simulink model "ModelOfLikeTheWholeThing"  (R2017b)
settings: Solver=ode8  StartTime=0.0  StopTime=5  FixedStep=0.01  RelTol=1e-3
InitFcn:
  | ra = 4;
  | jm = 0.0000218;
  | rm = 0.7/100;
  | dsm = 62.892;
  | kt = 0.138;
  | ke = kt;
  | ms = 0.93;
  | hl = 1.5 / 100;
  | Lr = 24.1 / 100;
  | Lcm = hl / 2 + Lr;
  | ml =0.182;
  | mr = 0.085;
  | rl = 20.125 / 1000;
  | Jp =1/3 * mr * Lr^2 + 1/2*ml*rl^2 + ml * Lcm ^ 2;
  | Dp = 0.007;
  | g = 9.82;
StartFcn:
  | ra = 4;
  | jm = 0.0000218;
  | rm = 0.7/100;
  | dsm = 62.892;
  | kt = 0.138;
  | ke = kt;
  | ms = 0.93;
settings Model: Creator=labadmin  LastModifiedBy=labadmin
settings RTWCC: SystemTargetFile=sldrt.tlc  TemplateMakefile=sldrt.tmf  Description=Simulink Desktop Real-Time  RTWCompilerOptimization=on
settings CodeAppCC: MaxIdLength=95
settings SimulinkDesktopRealTimeCC: TargetPreCompLibLocation=C:\Program Files\MATLAB\R2017b\toolbox\sldrt\lib\win64

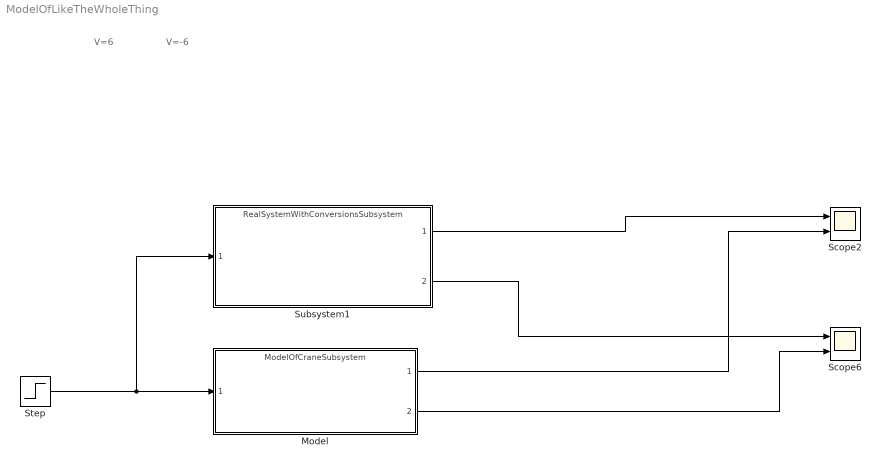
== system ModelOfLikeTheWholeThing ==
  note: V=6
  note: V=-6
  Model : ModelReference  ModelNameDialog=ModelOfCraneSubsystem.slx  SimulationMode=Normal  ModelReferenceVersion=1.4
  Scope2 : Scope  NumInputPorts=2
  Scope6 : Scope  NumInputPorts=2
  Step : Step  Time=2.5  After=0  SampleTime=0
  Subsystem1 : ModelReference  ModelNameDialog=RealSystemWithConversionsSubsystem  SimulationMode=Normal  ModelReferenceVersion=1.11
  wires:
  Step/1 -> Subsystem1/1, Model/1
  Model/1 -> Scope2/2
  Model/2 -> Scope6/2
  Subsystem1/1 -> Scope2/1
  Subsystem1/2 -> Scope6/1
